simulink model "pidsg"  (R2021a)
settings: Solver=VariableStepAuto  StartTime=0.0  StopTime=0.15  RelTol=1e-3
values from neighbouring files (symbols this model uses):
  aiw_G = 1    [pid_modelcomp_v1_0_setup.m]    (also in pid_sysgen_v1_0_setup.m)
  f_filter = SampleRate/Rr    (= 500)    [pid_modelcomp_v1_0_setup.m]    (also in pid_sysgen_v1_0_setup.m = 5000)
  FPGA_CLK_MHZ = 125    [pid_modelcomp_v1_0_setup.m]    (also in pid_sysgen_v1_0_setup.m)
  G1D = round(G1D*2^32)/2^32    [pid_modelcomp_v1_0_setup.m]    (also in pid_sysgen_v1_0_setup.m = 0.995012468828)
  G2D = round(G2D*2^7)/2^7    [pid_modelcomp_v1_0_setup.m]    (also in pid_sysgen_v1_0_setup.m = 349.163690773)
  Gi = round(Gi*2^25)/2^25    [pid_modelcomp_v1_0_setup.m]    (also in pid_sysgen_v1_0_setup.m = 2.5e-07)
  input_threshold = 0.0    (= 0)    [pid_modelcomp_v1_0_setup.m]    (also in pid_sysgen_v1_0_setup.m)
  kd = Gd*Ts/2    (= 0)    [pid_modelcomp_v1_0_setup.m]    (also in pid_sysgen_v1_0_setup.m = 0.07000732)
  ki = 2*Gi/Ts    (= 0)    [pid_modelcomp_v1_0_setup.m]    (also in pid_sysgen_v1_0_setup.m = 0.5)
  kp = round(kp*2^23)/2^23    [pid_modelcomp_v1_0_setup.m]    (also in pid_sysgen_v1_0_setup.m = 1.30000305)
  max_control = 0.9    [pid_modelcomp_v1_0_setup.m]    (also in pid_sysgen_v1_0_setup.m)
  SampleRate = 100.e3    (= 100000)    [pid_modelcomp_v1_0_setup.m]    (also in pid_sysgen_v1_0_setup.m = 1000000)
  Ts = 1/SampleRate    (= 1e-05)    [pid_modelcomp_v1_0_setup.m]    (also in pid_sysgen_v1_0_setup.m = 1e-06)
  VHDL_latency_cycles = 2    [pid_sysgen_v1_0_setup.m]
undefined symbols (not defined in the file or in its folder): xc7z030sbg485
libraries: hdlBasic x72, slpidlib x2, hdlUtilities x1, vmcUtilities x1
settings Model: Creator=osboxes  LastModifiedBy=valbas
settings SolverCC: AlgebraicLoopSolver=TrustRegion
settings DebuggingCC: SFMachineParentedDataDiag=warning

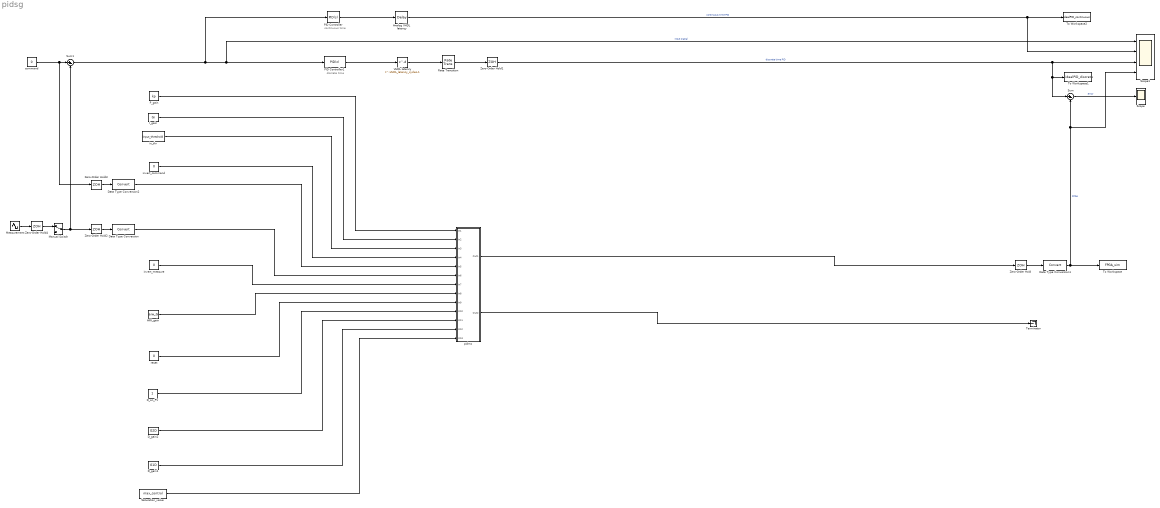
== system pidsg ==
  note: continuous time
  note: discrete time
  AIW_gain : Constant  Value=aiw_G  OutDataTypeStr=fixdt(1,32,30)  SampleTime=1/(FPGA_CLK_MHZ*1.e6)
  Analog VHDL latency : TransportDelay  DelayTime=VHDL_latency_cycles*Ts
  D_gain1 : Constant  Value=G1D  OutDataTypeStr=double  SampleTime=1/(FPGA_CLK_MHZ*1.e6)
  D_gain2 : Constant  Value=G2D  OutDataTypeStr=double  SampleTime=1/(FPGA_CLK_MHZ*1.e6)
  D_on_PV : Constant  OutDataTypeStr=boolean  SampleTime=1/(FPGA_CLK_MHZ*1.e6)
  Data Type Conversion : DataTypeConversion
  Data Type Conversion1 : DataTypeConversion
  Data Type Conversion2 : DataTypeConversion
  I_gain : Constant  Value=Gi  OutDataTypeStr=double  SampleTime=1/(FPGA_CLK_MHZ*1.e6)
  Manual Switch : ManualSwitch
  Measurement : Sin  Amplitude=0.01  Frequency=2*pi*21  Phase=0*pi  SampleTime=0
  PID Controller : slpidlib/PID Controller  Controller=PID  Form=Parallel  TimeDomain=Continuous-time  UseExternalTs=off  SampleTime=-1  IntegratorMethod=Forward Euler  FilterMethod=Forward Euler  ControllerParametersSource=internal  P=kp  I=ki  D=kd  UseFilter=on  N=f_filter  TunerSelectOption=Transfer Function Based (PID Tuner App)  InitialConditionSource=internal  InitialConditionForIntegrator=0  InitialConditionForFilter=0  DifferentiatorICPrevScaledInput=0  ExternalReset=none  TrackingMode=off  Kt=1  LimitOutput=off  SatLimitsSource=internal  UpperSaturationLimit=inf  LowerSaturationLimit=-inf  LinearizeAsGain=on  AntiWindupMode=none  Kb=1  POutMin=[]  POutMax=[]  IOutMin=[]  IOutMax=[]  DOutMin=[]  DOutMax=[]  NOutMin=[]  NOutMax=[]  SumOutMin=[]  SumOutMax=[]  SaturationOutMin=[]  SaturationOutMax=[]  PParamMin=[]  PParamMax=[]  IParamMin=[]  IParamMax=[]  DParamMin=[]  DParamMax=[]  NParamMin=[]  NParamMax=[]  KbParamMin=[]  KbParamMax=[]  KtParamMin=[]  KtParamMax=[]  KbOutMin=[]  KbOutMax=[]  KtOutMin=[]  KtOutMax=[]  IntegratorOutMin=[]  IntegratorOutMax=[]  FilterOutMin=[]  FilterOutMax=[]  SumI1OutMin=[]  SumI1OutMax=[]  SumI2OutMin=[]  SumI2OutMax=[]  SumI3OutMin=[]  SumI3OutMax=[]  SumI4OutMin=[]  SumI4OutMax=[]  SumDOutMin=[]  SumDOutMax=[]  DifferentiatorOutMin=[]  DifferentiatorOutMax=[]  FilterDiffOutCoefMin=[]  FilterDiffOutCoefMax=[]  ReciprocalOutMin=[]  ReciprocalOutMax=[]  SumDenOutMin=[]  SumDenOutMax=[]  SumNumOutMin=[]  SumNumOutMax=[]  DivideOutMin=[]  DivideOutMax=[]  UdiffTsProdOutMin=[]  UdiffTsProdOutMax=[]  NTsProdOutMin=[]  NTsProdOutMax=[]  UintegralTsProdOutMin=[]  UintegralTsProdOutMax=[]  UngainTsProdOutMin=[]  UngainTsProdOutMax=[]  IntegratorContinuousStateAttributes=''  IntegratorStateMustResolveToSignalObject=off  IntegratorRTWStateStorageClass=Auto  FilterContinuousStateAttributes=''  FilterStateMustResolveToSignalObject=off  FilterRTWStateStorageClass=Auto  ParallelPVariant=InternalParameters  IdealPVariant=Disabled  IVariant=InternalParameters  DVariant=InternalParameters  IntegratorVariant=Continuous  SatVariant=Disabled  AWVariant=Passthrough  PCopyVariant=Disabled  TRVariant=Disabled  FdbkBlocksVariant=Forward  IdealPFdbkVariant=Disabled  SatFdbkVariant=Disabled  DerivativeFilterVariant=ContFilter  NVariant=InternalParameters  NCopyVariant=Disabled  FilterICVariant=InternalICsFilter  IntegratorICVariant=InternalICs  ExternalResetVariant=Disabled  TRSumVariant=Passthrough  SumFdbkVariant=Disabled  SumVariant=Sum_PID  TsampFilterVariant=InternalTs  TsampNgainVariant=Passthrough  TsampIntegralVariant=Passthrough  ExternalSaturationOutDataTypeStr=Inherit: Same as second input
  PID Controller1 : slpidlib/PID Controller  Controller=PID  Form=Parallel  TimeDomain=Discrete-time  UseExternalTs=off  SampleTime=Ts  IntegratorMethod=Trapezoidal  FilterMethod=Trapezoidal  ControllerParametersSource=internal  P=kp  I=ki  D=kd  UseFilter=on  N=f_filter  TunerSelectOption=Transfer Function Based (PID Tuner App)  InitialConditionSource=internal  InitialConditionForIntegrator=0  InitialConditionForFilter=0  DifferentiatorICPrevScaledInput=0  ExternalReset=none  TrackingMode=off  Kt=1  LimitOutput=on  SatLimitsSource=internal  UpperSaturationLimit=max_control  LowerSaturationLimit=-max_control  LinearizeAsGain=on  AntiWindupMode=back-calculation  Kb=aiw_G*ki  POutMin=[]  POutMax=[]  IOutMin=[]  IOutMax=[]  DOutMin=[]  DOutMax=[]  NOutMin=[]  NOutMax=[]  SumOutMin=[]  SumOutMax=[]  SaturationOutMin=[]  SaturationOutMax=[]  PParamMin=[]  PParamMax=[]  IParamMin=[]  IParamMax=[]  DParamMin=[]  DParamMax=[]  NParamMin=[]  NParamMax=[]  KbParamMin=[]  KbParamMax=[]  KtParamMin=[]  KtParamMax=[]  KbOutMin=[]  KbOutMax=[]  KtOutMin=[]  KtOutMax=[]  IntegratorOutMin=[]  IntegratorOutMax=[]  FilterOutMin=[]  FilterOutMax=[]  SumI1OutMin=[]  SumI1OutMax=[]  SumI2OutMin=[]  SumI2OutMax=[]  SumI3OutMin=[]  SumI3OutMax=[]  SumI4OutMin=[]  SumI4OutMax=[]  SumDOutMin=[]  SumDOutMax=[]  DifferentiatorOutMin=[]  DifferentiatorOutMax=[]  FilterDiffOutCoefMin=[]  FilterDiffOutCoefMax=[]  ReciprocalOutMin=[]  ReciprocalOutMax=[]  SumDenOutMin=[]  SumDenOutMax=[]  SumNumOutMin=[]  SumNumOutMax=[]  DivideOutMin=[]  DivideOutMax=[]  UdiffTsProdOutMin=[]  UdiffTsProdOutMax=[]  NTsProdOutMin=[]  NTsProdOutMax=[]  UintegralTsProdOutMin=[]  UintegralTsProdOutMax=[]  UngainTsProdOutMin=[]  UngainTsProdOutMax=[]  IntegratorContinuousStateAttributes=''  IntegratorStateMustResolveToSignalObject=off  IntegratorRTWStateStorageClass=Auto  FilterContinuousStateAttributes=''  FilterStateMustResolveToSignalObject=off  FilterRTWStateStorageClass=Auto  ParallelPVariant=InternalParameters  IdealPVariant=Disabled  IVariant=InternalParameters  DVariant=InternalParameters  IntegratorVariant=Discrete  SatVariant=Enabled  AWVariant=BackCalculation  PCopyVariant=Disabled  TRVariant=Disabled  FdbkBlocksVariant=Feedback  IdealPFdbkVariant=Passthrough  SatFdbkVariant=Enabled  DerivativeFilterVariant=TrapezoidalFilter  NVariant=InternalParameters  NCopyVariant=InternalParameters  FilterICVariant=InternalICsFilter  IntegratorICVariant=InternalICs  ExternalResetVariant=Disabled  TRSumVariant=Passthrough  SumFdbkVariant=Enabled  SumVariant=Sum_PID  TsampFilterVariant=InternalTs  TsampNgainVariant=Passthrough  TsampIntegralVariant=Passthrough  ExternalSaturationOutDataTypeStr=Inherit: Same as second input
  P_gain : Constant  Value=kp  OutDataTypeStr=double  SampleTime=1/(FPGA_CLK_MHZ*1.e6)
  Rate Transition : RateTransition  OutPortSampleTime=1/(FPGA_CLK_MHZ*1.e6)
  Saturation_value : Constant  Value=max_control  OutDataTypeStr=fixdt(1,32,30)  SampleTime=1/(FPGA_CLK_MHZ*1.e6)
  Scope : Scope
  Scope1 : Scope  NumInputPorts=4
  Sum : Sum  Inputs=|+-
  Sum1 : Sum  Inputs=|+-
  Terminator : Terminator
  To Workspace : ToWorkspace  VariableName=FPGA_sim  SampleTime=-1
      settings: Decimation=125
  To Workspace1 : ToWorkspace  VariableName=idealPID_discrete  SaveFormat=Timeseries  SampleTime=-1
      settings: Decimation=125
  To Workspace2 : ToWorkspace  VariableName=idealPID_continuous  SaveFormat=Timeseries  SampleTime=-1
  VHDL latency : Delay  DelayLength=VHDL_latency_cycles-1
  Zero-Order Hold{,1..3} (4 alike) : ZeroOrderHold  SampleTime=1/(FPGA_CLK_MHZ*1.e6)
  Zero-Order Hold4 : ZeroOrderHold  SampleTime=Ts
  command : Constant  Value=0  OutDataTypeStr=double  SampleTime=0
  in_thr : Constant  Value=input_threshold  OutDataTypeStr=fixdt(1,32,30)  SampleTime=1/(FPGA_CLK_MHZ*1.e6)
  invert_command : Constant  Value=0  OutDataTypeStr=boolean  SampleTime=1/(FPGA_CLK_MHZ*1.e6)
  invert_measure : Constant  Value=0  OutDataTypeStr=boolean  SampleTime=1/(FPGA_CLK_MHZ*1.e6)
  pidmc : Subsystem
  reset : Constant  Value=0  OutDataTypeStr=boolean  SampleTime=1/(FPGA_CLK_MHZ*1.e6)
  wires:
  Data Type Conversion1/1 -> To Workspace/1, Scope1/4, Sum/2  "FPGA"
  PID Controller1/1 -> VHDL latency/1
  command/1 -> Zero-Order Hold3/1, Sum1/1
  PID Controller/1 -> Analog VHDL latency/1
  Analog VHDL latency/1 -> To Workspace2/1, Scope1/2  "continuous time PID"
  Sum/1 -> Scope/1  "error"
  Sum1/1 -> Scope1/1, PID Controller1/1, PID Controller/1  "input signal"
  VHDL latency/1 -> Rate Transition/1
  Zero-Order Hold/1 -> Data Type Conversion1/1
  Zero-Order Hold1/1 -> To Workspace1/1, Sum/1, Scope1/3  "discrete time PID"
  Zero-Order Hold2/1 -> Data Type Conversion/1
  Zero-Order Hold3/1 -> Data Type Conversion2/1
  Rate Transition/1 -> Zero-Order Hold1/1
  Manual Switch/1 -> Sum1/2, Zero-Order Hold2/1
  Measurement/1 -> Zero-Order Hold4/1
  Zero-Order Hold4/1 -> Manual Switch/1
  P_gain/1 -> pidmc/1(In1)
  I_gain/1 -> pidmc/2(In2)
  in_thr/1 -> pidmc/3(In3)
  invert_command/1 -> pidmc/4(In4)
  Data Type Conversion2/1 -> pidmc/5(In5)
  Data Type Conversion/1 -> pidmc/6(In6)
  invert_measure/1 -> pidmc/7(In7)
  AIW_gain/1 -> pidmc/8(In8)
  reset/1 -> pidmc/9(In9)
  D_on_PV/1 -> pidmc/10(In10)
  D_gain2/1 -> pidmc/11(In11)
  D_gain1/1 -> pidmc/12(In12)
  Saturation_value/1 -> pidmc/13(In13)
  pidmc/1(Out1) -> Zero-Order Hold/1
  pidmc/2(Out2) -> Terminator/1

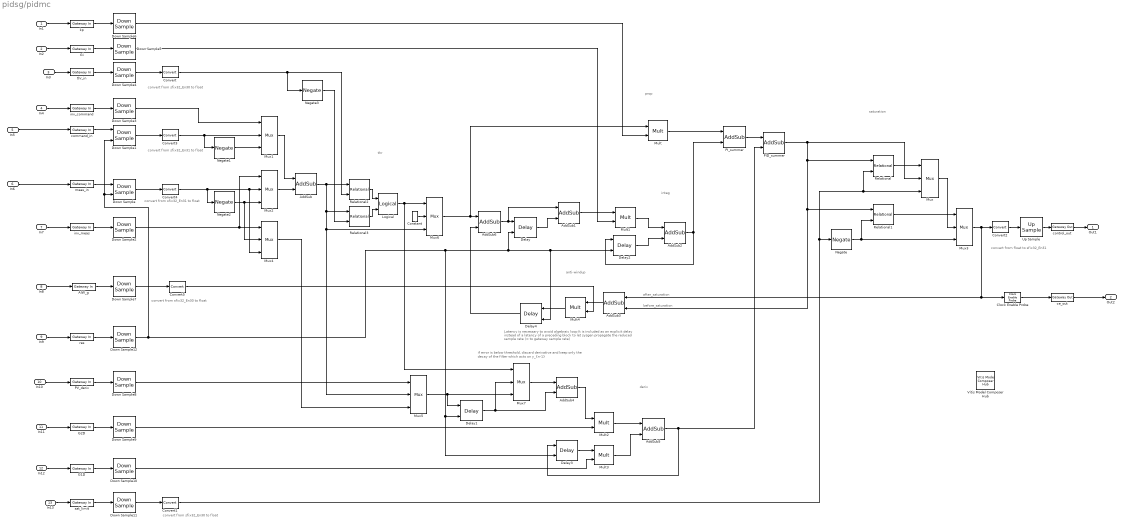
== system pidsg/pidmc ==
  note: saturation
  note: convert from sfix32_En30 to float
  note: anti-windup
  note: before_saturation
  note: integ
  note: thr
  note: prop
  note: if error is below threshold, discard derivative and keep only
      | the decay of the filter which acts on y_{n-1}
  note: Latency is necessary to avoid algebraic loop
      | It is included as an explicit delay instead of a latency of a preceding block
      | to let sysgen propagate the reduced sample rate (= to gateway sample rate)
  note: convert from float to sfix32_En31
  note: convert from sfix32_En30 to float
  note: after_saturation
  note: convert from sfix32_En31 to float
  note: convert from sfix32_En31 to float
  note: deriv
  note: convert from sfix32_En30 to float
  In1 : Inport
  In2 : Inport  Port=2
  In3 : Inport  Port=3
  In4 : Inport  Port=4
  In5 : Inport  Port=5
  In6 : Inport  Port=6
  In7 : Inport  Port=7
  In8 : Inport  Port=8
  In9 : Inport  Port=9
  In10 : Inport  Port=10
  In11 : Inport  Port=11
  In12 : Inport  Port=12
  In13 : Inport  Port=13
  AIW_g : hdlBasic/Gateway In  gui_display_data_type=Fixed-point  arith_type=Signed (2's comp)  n_bits=32  bin_pt=30  preci_type=Single  exp_width=8  frac_width=24  rows=1  columns=1  quantization="Round  (unbiased: +/- Inf)"  overflow=Saturate  period=1/(FPGA_CLK_MHZ*1.e6)  UseAsADC=off  ADCChannel='1'  interface=None  automatic_assignment=on  address_offset=hex2dec('00')  intf_name=''  intf_description=''  default_value=0  timing_constraint=None  locs_specified=off  LOCs={}  io_standard={}  inherit_from_input=off  hdl_port=on  XmcBlockStatus=1  maskContainerNames=group4  block_type=gatewayin  block_config=sysgen:gateway_in_config  block_width_w=590  block_height_w=620  block_width=640  block_height=850
  AddSub : hdlBasic/AddSub  mode=Subtraction  use_carryin=off  use_carryout=off  en=off  latency=0  precision=Full  arith_type=Unsigned  n_bits=16  bin_pt=14  quantization=Truncate  overflow=Wrap  use_behavioral_HDL=off  hw_selection=Fabric  pipelined=off  XmcBlockStatus=1  maskContainerNames=tabcontainer1  block_type=addsub  block_config=sysgen:Addsub_config
  AddSub{1..2,5..6} (4 alike) : hdlBasic/AddSub  mode=Addition  use_carryin=off  use_carryout=off  en=off  latency=0  precision=Full  arith_type=Unsigned  n_bits=16  bin_pt=14  quantization=Truncate  overflow=Wrap  use_behavioral_HDL=off  hw_selection=Fabric  pipelined=off  XmcBlockStatus=1  maskContainerNames=tabcontainer1  block_type=addsub  block_config=sysgen:Addsub_config
  AddSub3 : hdlBasic/AddSub  mode=Subtraction  use_carryin=off  use_carryout=off  en=off  latency=0  precision=Full  arith_type=Unsigned  n_bits=16  bin_pt=14  quantization=Truncate  overflow=Wrap  use_behavioral_HDL=off  hw_selection=Fabric  pipelined=off  XmcBlockStatus=1  maskContainerNames=tabcontainer1  block_type=addsub  block_config=sysgen:Addsub_config
  AddSub4 : hdlBasic/AddSub  mode=Subtraction  use_carryin=off  use_carryout=off  en=off  latency=0  precision=Full  arith_type=Unsigned  n_bits=16  bin_pt=14  quantization=Truncate  overflow=Wrap  use_behavioral_HDL=off  hw_selection=Fabric  pipelined=off  XmcBlockStatus=1  maskContainerNames=tabcontainer1  block_type=addsub  block_config=sysgen:Addsub_config
  Clock Enable Probe : hdlUtilities/Clock Enable Probe  inherit_constraints=on  XmcBlockStatus=1  maskContainerNames=group1  block_type=ceprobe  block_config=sysgen:CEProbe_config
  Constant : hdlBasic/Constant  const=0  gui_display_data_type=Floating-point  arith_type=Floating-point  n_bits=16  bin_pt=14  preci_type=Single  exp_width=8  frac_width=24  explicit_period=off  period=1  XmcBlockStatus=1  maskContainerNames=tabcontainer1  block_type=constant  block_config=sysgen:Constant_config
  Convert{,1,3..5} (5 alike) : hdlBasic/Convert  gui_display_data_type=Floating-point  arith_type=Floating-point  n_bits=16  bin_pt=14  float_type=Single  exp_bits=8  fraction_bits=24  quantization=Truncate  overflow=Wrap  en=off  latency=0  pipeline=off  XmcBlockStatus=1  maskContainerNames=group2  block_type=convert  block_config=sysgen:Convert_config  block_width=595  block_height=885
  Convert2 : hdlBasic/Convert  gui_display_data_type=Fixed-point  arith_type=Signed (2's comp)  n_bits=32  bin_pt=31  float_type=Single  exp_bits=8  fraction_bits=24  quantization="Round  (unbiased: +/- Inf)"  overflow=Saturate  en=off  latency=0  pipeline=off  XmcBlockStatus=1  maskContainerNames=group2  block_type=convert  block_config=sysgen:Convert_config  block_width=595  block_height=885
  Delay{,1..4} (5 alike) : hdlBasic/Delay  rst=on  en=off  latency=1  reg_retiming=off  XmcBlockStatus=1  maskContainerNames=group1  block_type=delay  block_config=sysgen:Delay_config
  Down Sample : hdlBasic/Down Sample  sample_ratio=FPGA_CLK_MHZ*1.e6/SampleRate  sample_phase="Last Value of Frame  (most efficient)"  en=off  rst=on  latency=1  XmcBlockStatus=1  maskContainerNames=group1  block_type=dsamp  block_config=sysgen:Downsample_config
  Down Sample1 : hdlBasic/Down Sample  sample_ratio=FPGA_CLK_MHZ*1.e6/SampleRate  sample_phase="Last Value of Frame  (most efficient)"  en=off  rst=on  latency=1  XmcBlockStatus=1  maskContainerNames=group1  block_type=dsamp  block_config=sysgen:Downsample_config
  Down Sample{2..12} (11 alike) : hdlBasic/Down Sample  sample_ratio=FPGA_CLK_MHZ*1.e6/SampleRate  sample_phase="Last Value of Frame  (most efficient)"  en=off  rst=off  latency=1  XmcBlockStatus=1  maskContainerNames=group1  block_type=dsamp  block_config=sysgen:Downsample_config
  G1D : hdlBasic/Gateway In  gui_display_data_type=Floating-point  arith_type=Floating-point  n_bits=16  bin_pt=14  preci_type=Single  exp_width=8  frac_width=24  rows=1  columns=1  quantization="Round  (unbiased: +/- Inf)"  overflow=Saturate  period=1/(FPGA_CLK_MHZ*1.e6)  UseAsADC=off  ADCChannel='1'  interface=None  automatic_assignment=on  address_offset=hex2dec('00')  intf_name=''  intf_description=''  default_value=0  timing_constraint=None  locs_specified=off  LOCs={}  io_standard={}  inherit_from_input=off  hdl_port=on  XmcBlockStatus=1  maskContainerNames=group4  block_type=gatewayin  block_config=sysgen:gateway_in_config  block_width_w=590  block_height_w=620  block_width=640  block_height=850
  G2D : hdlBasic/Gateway In  gui_display_data_type=Floating-point  arith_type=Floating-point  n_bits=16  bin_pt=14  preci_type=Single  exp_width=8  frac_width=24  rows=1  columns=1  quantization="Round  (unbiased: +/- Inf)"  overflow=Saturate  period=1/(FPGA_CLK_MHZ*1.e6)  UseAsADC=off  ADCChannel='1'  interface=None  automatic_assignment=on  address_offset=hex2dec('00')  intf_name=''  intf_description=''  default_value=0  timing_constraint=None  locs_specified=off  LOCs={}  io_standard={}  inherit_from_input=off  hdl_port=on  XmcBlockStatus=1  maskContainerNames=group4  block_type=gatewayin  block_config=sysgen:gateway_in_config  block_width_w=590  block_height_w=620  block_width=640  block_height=850
  Gi : hdlBasic/Gateway In  gui_display_data_type=Floating-point  arith_type=Floating-point  n_bits=16  bin_pt=14  preci_type=Single  exp_width=8  frac_width=24  rows=1  columns=1  quantization="Round  (unbiased: +/- Inf)"  overflow=Saturate  period=1/(FPGA_CLK_MHZ*1.e6)  UseAsADC=off  ADCChannel='1'  interface=None  automatic_assignment=on  address_offset=hex2dec('00')  intf_name=''  intf_description=''  default_value=0  timing_constraint=None  locs_specified=off  LOCs={}  io_standard={}  inherit_from_input=off  hdl_port=on  XmcBlockStatus=1  maskContainerNames=group4  block_type=gatewayin  block_config=sysgen:gateway_in_config  block_width_w=590  block_height_w=620  block_width=640  block_height=850
  Logical : hdlBasic/Logical  logical_function=OR  inputs=2  en=off  latency=0  precision=Full  arith_type=Unsigned  n_bits=16  bin_pt=0  align_bp=on  overflow=[]  quantization=[]  XmcBlockStatus=1  maskContainerNames=tabcontainer1  block_type=logical  block_config=sysgen:Logical_config
  Mult{,1..4} (5 alike) : hdlBasic/Mult  precision=Full  arith_type="Signed  (2's comp)"  n_bits=16  bin_pt=14  quantization=Truncate  overflow=Wrap  en=off  latency=0  use_behavioral_HDL=off  opt=Speed  use_embedded=on  optimum_pipeline=off  pipeline=on  use_rpm=on  placement_style=Triangular  XmcBlockStatus=1  maskContainerNames=group1  block_type=mult  block_config=sysgen:Mult_config  block_width=598  block_height=876
  Mux{,1..7} (8 alike) : hdlBasic/Mux  inputs=2  en=off  latency=0  precision=Full  arith_type=Unsigned  n_bits=16  bin_pt=14  quantization=Truncate  overflow=Wrap  XmcBlockStatus=1  maskContainerNames=tabcontainer1  block_type=mux  block_config=sysgen:Mux_config
  Negate{,1..3} (4 alike) : hdlBasic/Negate  precision=Full  arith_type=Unsigned  n_bits=16  bin_pt=14  quantization=Truncate  overflow=Wrap  en=off  latency=0  XmcBlockStatus=1  maskContainerNames=tabcontainer1  block_type=negate  block_config=sysgen:Negate_config
  PID_summer : hdlBasic/AddSub  mode=Addition  use_carryin=off  use_carryout=off  en=off  latency=0  precision=Full  arith_type=Unsigned  n_bits=16  bin_pt=14  quantization=Truncate  overflow=Wrap  use_behavioral_HDL=off  hw_selection=Fabric  pipelined=off  XmcBlockStatus=1  maskContainerNames=tabcontainer1  block_type=addsub  block_config=sysgen:Addsub_config
  PI_summer : hdlBasic/AddSub  mode=Addition  use_carryin=off  use_carryout=off  en=off  latency=0  precision=Full  arith_type=Unsigned  n_bits=16  bin_pt=14  quantization=Truncate  overflow=Wrap  use_behavioral_HDL=off  hw_selection=Fabric  pipelined=off  XmcBlockStatus=1  maskContainerNames=tabcontainer1  block_type=addsub  block_config=sysgen:Addsub_config
  PV_deriv : hdlBasic/Gateway In  gui_display_data_type=Boolean  arith_type=Boolean  n_bits=16  bin_pt=14  preci_type=Single  exp_width=8  frac_width=24  rows=1  columns=1  quantization="Round  (unbiased: +/- Inf)"  overflow=Saturate  period=1/(FPGA_CLK_MHZ*1.e6)  UseAsADC=off  ADCChannel='1'  interface=None  automatic_assignment=on  address_offset=hex2dec('00')  intf_name=''  intf_description=''  default_value=0  timing_constraint=None  locs_specified=off  LOCs={}  io_standard={}  inherit_from_input=off  hdl_port=on  XmcBlockStatus=1  maskContainerNames=group4  block_type=gatewayin  block_config=sysgen:gateway_in_config  block_width_w=590  block_height_w=620  block_width=640  block_height=850
  Relational : hdlBasic/Relational  mode=a>b  op_type=Bool  en=off  latency=0  XmcBlockStatus=1  maskContainerNames=tabcontainer1  block_type=relational  block_config=sysgen:Relational_config
  Relational1 : hdlBasic/Relational  mode=a<b  op_type=Bool  en=off  latency=0  XmcBlockStatus=1  maskContainerNames=tabcontainer1  block_type=relational  block_config=sysgen:Relational_config
  Relational2 : hdlBasic/Relational  mode=a>b  op_type=Bool  en=off  latency=0  XmcBlockStatus=1  maskContainerNames=tabcontainer1  block_type=relational  block_config=sysgen:Relational_config
  Relational3 : hdlBasic/Relational  mode=a<b  op_type=Bool  en=off  latency=0  XmcBlockStatus=1  maskContainerNames=tabcontainer1  block_type=relational  block_config=sysgen:Relational_config
  Up Sample : hdlBasic/Up Sample  sample_ratio=FPGA_CLK_MHZ*1.e6/SampleRate  copy_samples=on  en=off  latency=1  XmcBlockStatus=1  maskContainerNames=group1  block_type=usamp  block_config=sysgen:Upsample_config
  Vitis Model Composer Hub : vmcUtilities/Vitis Model Composer Hub  Tag=genX  CodeGeneration=off  TargetDirectory=./code  ExportType=System Generator  IpVendor=xilinx.com  IpLibrary=hls  IpVersion=1.0  IpHWLanguage=Verilog  AieCompilerOptions={}  CreateTestbench=off  TestbenchStackSize=10  RunAieSim=off  AieSimTimeout=50000  RunAieSimProfiling=off  LaunchVitisAnalyzer=off  PlotOutput=off  RunX86Sim=off  X86SimTimeout=10  GenHwImage=off  PlatformType=Not Specified  HwSystemType=Baremetal  HwValidationTarget=hw  ProjDevice=xc7z030sbg485-1  ProjDevicePart=xc7z030sbg485-1  SamplePeriod=-1  ClockFrequency=200  DataPathParallelism=1  xilinxfamily=zynq  part=xc7z030  speed=-1  package=sbg485  directory=./netlist  testbench=off  incr_netlist=off  synthesis_tool=Vivado  clock_wrapper=Clock Enables  dbl_ovrd=According to Block Masks  dcm_input_clock_period=10  sysclk_period=1.e3/FPGA_CLK_MHZ  simulink_period=1/(FPGA_CLK_MHZ*1.e6)  eval_field=0  IPInfoJsonString="{\"HDLSubsystem\":{\"SubsystemName\":\"pidmc\",\"IPName\":\"pidmc\",\"IPLibrary\":\"Panda_ModelComp\",\"IPVendor\":\"MaxIV\",\"IPVersion\":\"1.0\"}}"
  ce_out : hdlBasic/Gateway Out  inherit_from_input=on  hdl_port=on  rows=1  columns=1  UseAsDAC=off  DACChannel='1'  interface=None  automatic_assignment=on  address_offset=hex2dec('00')  intf_name=''  intf_description=''  timing_constraint=Data Rate  locs_specified=off  LOCs={}  io_standard={}  XmcBlockStatus=1  maskContainerNames=group4  block_type=gatewayout  block_config=sysgen:gateway_out_config  block_width_w=590  block_height_w=620  block_width=620  block_height=750
  command_in : hdlBasic/Gateway In  gui_display_data_type=Fixed-point  arith_type=Signed (2's comp)  n_bits=32  bin_pt=31  preci_type=Single  exp_width=8  frac_width=24  rows=1  columns=1  quantization="Round  (unbiased: +/- Inf)"  overflow=Saturate  period=1/(FPGA_CLK_MHZ*1.e6)  UseAsADC=off  ADCChannel='1'  interface=None  automatic_assignment=on  address_offset=hex2dec('00')  intf_name=''  intf_description=''  default_value=0  timing_constraint=None  locs_specified=off  LOCs={}  io_standard={}  inherit_from_input=off  hdl_port=on  XmcBlockStatus=1  maskContainerNames=group4  block_type=gatewayin  block_config=sysgen:gateway_in_config  block_width_w=590  block_height_w=620  block_width=640  block_height=850
  control_out : hdlBasic/Gateway Out  inherit_from_input=on  hdl_port=on  rows=1  columns=1  UseAsDAC=off  DACChannel='1'  interface=None  automatic_assignment=on  address_offset=hex2dec('00')  intf_name=''  intf_description=''  timing_constraint=Data Rate  locs_specified=off  LOCs={}  io_standard={}  XmcBlockStatus=1  maskContainerNames=group4  block_type=gatewayout  block_config=sysgen:gateway_out_config  block_width_w=590  block_height_w=620  block_width=620  block_height=750
  inv_command : hdlBasic/Gateway In  gui_display_data_type=Boolean  arith_type=Boolean  n_bits=16  bin_pt=14  preci_type=Single  exp_width=8  frac_width=24  rows=1  columns=1  quantization="Round  (unbiased: +/- Inf)"  overflow=Saturate  period=1/(FPGA_CLK_MHZ*1.e6)  UseAsADC=off  ADCChannel='1'  interface=None  automatic_assignment=on  address_offset=hex2dec('00')  intf_name=''  intf_description=''  default_value=0  timing_constraint=None  locs_specified=off  LOCs={}  io_standard={}  inherit_from_input=off  hdl_port=on  XmcBlockStatus=1  maskContainerNames=group4  block_type=gatewayin  block_config=sysgen:gateway_in_config  block_width_w=590  block_height_w=620  block_width=640  block_height=850
  inv_meas : hdlBasic/Gateway In  gui_display_data_type=Boolean  arith_type=Boolean  n_bits=16  bin_pt=14  preci_type=Single  exp_width=8  frac_width=24  rows=1  columns=1  quantization="Round  (unbiased: +/- Inf)"  overflow=Saturate  period=1/(FPGA_CLK_MHZ*1.e6)  UseAsADC=off  ADCChannel='1'  interface=None  automatic_assignment=on  address_offset=hex2dec('00')  intf_name=''  intf_description=''  default_value=0  timing_constraint=None  locs_specified=off  LOCs={}  io_standard={}  inherit_from_input=off  hdl_port=on  XmcBlockStatus=1  maskContainerNames=group4  block_type=gatewayin  block_config=sysgen:gateway_in_config  block_width_w=590  block_height_w=620  block_width=640  block_height=850
  kp : hdlBasic/Gateway In  gui_display_data_type=Floating-point  arith_type=Floating-point  n_bits=16  bin_pt=14  preci_type=Single  exp_width=8  frac_width=24  rows=1  columns=1  quantization="Round  (unbiased: +/- Inf)"  overflow=Saturate  period=1/(FPGA_CLK_MHZ*1.e6)  UseAsADC=off  ADCChannel='1'  interface=None  automatic_assignment=on  address_offset=hex2dec('00')  intf_name=''  intf_description=''  default_value=0  timing_constraint=None  locs_specified=off  LOCs={}  io_standard={}  inherit_from_input=off  hdl_port=on  XmcBlockStatus=1  maskContainerNames=group4  block_type=gatewayin  block_config=sysgen:gateway_in_config  block_width_w=590  block_height_w=620  block_width=640  block_height=850
  meas_in : hdlBasic/Gateway In  gui_display_data_type=Fixed-point  arith_type=Signed (2's comp)  n_bits=32  bin_pt=31  preci_type=Single  exp_width=8  frac_width=24  rows=1  columns=1  quantization="Round  (unbiased: +/- Inf)"  overflow=Saturate  period=1/(FPGA_CLK_MHZ*1.e6)  UseAsADC=off  ADCChannel='1'  interface=None  automatic_assignment=on  address_offset=hex2dec('00')  intf_name=''  intf_description=''  default_value=0  timing_constraint=None  locs_specified=off  LOCs={}  io_standard={}  inherit_from_input=off  hdl_port=on  XmcBlockStatus=1  maskContainerNames=group4  block_type=gatewayin  block_config=sysgen:gateway_in_config  block_width_w=590  block_height_w=620  block_width=640  block_height=850
  res : hdlBasic/Gateway In  gui_display_data_type=Boolean  arith_type=Boolean  n_bits=16  bin_pt=14  preci_type=Single  exp_width=8  frac_width=24  rows=1  columns=1  quantization="Round  (unbiased: +/- Inf)"  overflow=Saturate  period=1/(FPGA_CLK_MHZ*1.e6)  UseAsADC=off  ADCChannel='1'  interface=None  automatic_assignment=on  address_offset=hex2dec('00')  intf_name=''  intf_description=''  default_value=0  timing_constraint=None  locs_specified=off  LOCs={}  io_standard={}  inherit_from_input=off  hdl_port=on  XmcBlockStatus=1  maskContainerNames=group4  block_type=gatewayin  block_config=sysgen:gateway_in_config  block_width_w=590  block_height_w=620  block_width=640  block_height=850
  sat_limit : hdlBasic/Gateway In  gui_display_data_type=Fixed-point  arith_type=Signed (2's comp)  n_bits=32  bin_pt=30  preci_type=Single  exp_width=8  frac_width=24  rows=1  columns=1  quantization="Round  (unbiased: +/- Inf)"  overflow=Saturate  period=1/(FPGA_CLK_MHZ*1.e6)  UseAsADC=off  ADCChannel='1'  interface=None  automatic_assignment=on  address_offset=hex2dec('00')  intf_name=''  intf_description=''  default_value=0  timing_constraint=None  locs_specified=off  LOCs={}  io_standard={}  inherit_from_input=off  hdl_port=on  XmcBlockStatus=1  maskContainerNames=group4  block_type=gatewayin  block_config=sysgen:gateway_in_config  block_width_w=590  block_height_w=620  block_width=640  block_height=850
  thr_in : hdlBasic/Gateway In  gui_display_data_type=Fixed-point  arith_type=Signed (2's comp)  n_bits=32  bin_pt=30  preci_type=Single  exp_width=8  frac_width=24  rows=1  columns=1  quantization="Round  (unbiased: +/- Inf)"  overflow=Saturate  period=1/(FPGA_CLK_MHZ*1.e6)  UseAsADC=off  ADCChannel='1'  interface=None  automatic_assignment=on  address_offset=hex2dec('00')  intf_name=''  intf_description=''  default_value=0  timing_constraint=None  locs_specified=off  LOCs={}  io_standard={}  inherit_from_input=off  hdl_port=on  XmcBlockStatus=1  maskContainerNames=group4  block_type=gatewayin  block_config=sysgen:gateway_in_config  block_width_w=590  block_height_w=620  block_width=640  block_height=850
  Out1 : Outport
  Out2 : Outport  Port=2
  wires:
  kp/1 -> Down Sample6/1
  Down Sample11/1 -> Convert1/1
  command_in/1 -> Down Sample1/1
  PV_deriv/1 -> Down Sample8/1
  Mult/1 -> PI_summer/1
  In12/1 -> G1D/1
  Down Sample10/1 -> Mult3/2
  AddSub1/1 -> Mult1/1
  PID_summer/1 -> Mux/2, AddSub3/2, Relational1/1, Relational/1
  G2D/1 -> Down Sample9/1
  Delay1/1 -> Mux7/2, AddSub4/2
  Down Sample5/1 -> Mult1/2
  AddSub5/1 -> PID_summer/2, Delay3/1
  Negate1/1 -> Mux1/3
  Negate/1 -> Mux3/3, Relational1/2
  PI_summer/1 -> PID_summer/1
  Convert2/1 -> Up Sample/1
  Mux4/1 -> Mux5/3
  Mult1/1 -> AddSub2/1
  Mux/1 -> Mux3/2
  Convert3/1 -> Negate1/1, Mux1/2
  inv_meas/1 -> Down Sample2/1
  control_out/1 -> Out1/1
  thr_in/1 -> Down Sample4/1
  In10/1 -> PV_deriv/1
  Mux7/1 -> AddSub4/1
  Down Sample2/1 -> Mux4/1, Mux2/1
  Relational3/1 -> Logical/2
  In13/1 -> sat_limit/1
  Convert4/1 -> Mux4/3, Mux2/2, Negate2/1
  Mux1/1 -> AddSub/1
  Down Sample12/1 -> Delay3/2, Delay1/2, Delay/2, Delay2/2, Delay4/2, Down Sample/2, Down Sample1/2
  In1/1 -> kp/1
  Convert1/1 -> Relational/2, Mux/3, Negate/1
  Down Sample4/1 -> Convert/1
  ce_out/1 -> Out2/1
  In11/1 -> G2D/1
  Down Sample7/1 -> Convert5/1
  Down Sample6/1 -> Mult/2
  In8/1 -> AIW_g/1
  Down Sample3/1 -> Mux1/1
  Gi/1 -> Down Sample5/1
  Relational/1 -> Mux/1
  Up Sample/1 -> control_out/1
  In7/1 -> inv_meas/1
  res/1 -> Down Sample12/1
  Mult4/1 -> Delay4/1
  Clock Enable Probe/1 -> ce_out/1
  Mux3/1 -> Convert2/1, Clock Enable Probe/1, AddSub3/1
  Down Sample9/1 -> Mult2/2
  AddSub4/1 -> Mult2/1
  Mux5/1 -> Mux7/3, Delay1/1
  Mux6/1 -> AddSub6/1, Mult/1
  Down Sample1/1 -> Convert3/1
  Constant/1 -> Mux6/2
  In2/1 -> Gi/1
  AddSub/1 -> Relational2/1, Relational3/1, Mux6/3, Mux5/2
  Convert/1 -> Negate3/1, Relational2/2
  Convert5/1 -> Mult4/2
  Logical/1 -> Mux7/1, Mux6/1
  AddSub2/1 -> Delay2/1, PI_summer/2
  Delay3/1 -> Mult3/1
  sat_limit/1 -> Down Sample11/1
  In5/1 -> command_in/1
  Down Sample/1 -> Convert4/1
  Delay2/1 -> AddSub2/2
  Mult3/1 -> AddSub5/2
  Mux2/1 -> AddSub/2
  Down Sample8/1 -> Mux5/1
  Relational1/1 -> Mux3/1
  inv_command/1 -> Down Sample3/1
  In4/1 -> inv_command/1
  In3/1 -> thr_in/1
  Delay4/1 -> AddSub6/2
  Mult2/1 -> AddSub5/1
  AddSub6/1 -> AddSub1/1, Delay/1
  Negate2/1 -> Mux4/2, Mux2/3
  AddSub3/1 -> Mult4/1
  Negate3/1 -> Relational3/2
  AIW_g/1 -> Down Sample7/1
  Relational2/1 -> Logical/1
  G1D/1 -> Down Sample10/1
  In9/1 -> res/1
  In6/1 -> meas_in/1
  meas_in/1 -> Down Sample/1
  Delay/1 -> AddSub1/2
